simulink model "Clase26112020"  (R2020b)
settings: Solver=VariableStepAuto  StartTime=0.0  StopTime=2  RelTol=1e-3
libraries: dspvision x2, commanapbnd3 x1
settings Model: Creator=fernando  LastModifiedBy=fernando

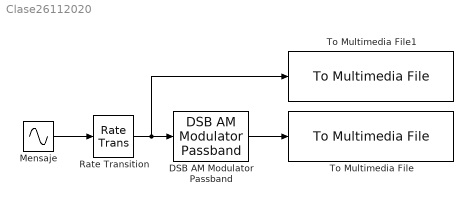
== system Clase26112020 ==
  DSB AM Modulator Passband : commanapbnd3/DSB AM Modulator Passband  Fc=10E3  Ph=0  Offset=1
      settings: SourceProductBaseCode=CM
  Mensaje : Sin  Frequency=2*pi*440  SampleTime=0
  Rate Transition : RateTransition  OutPortSampleTime=1/44100
  To Multimedia File : dspvision/To Multimedia File  outputFilename=SalidaModulada.wav  streamSelection=Audio only  videoCompressor=None (uncompressed)  audioCompressor=None (uncompressed)  imagePorts=Separate color signals  fileType=WAV  audioDatatype=16-bit integer  fourcc=RGB  videoQuality=75  mj2000CompFactor=10
  To Multimedia File1 : dspvision/To Multimedia File  outputFilename=SalidaNoModulada.wav  streamSelection=Audio only  videoCompressor=None (uncompressed)  audioCompressor=None (uncompressed)  imagePorts=Separate color signals  fileType=WAV  audioDatatype=16-bit integer  fourcc=RGB  videoQuality=75  mj2000CompFactor=10
  wires:
  Mensaje/1 -> Rate Transition/1
  Rate Transition/1 -> To Multimedia File1/1, DSB AM Modulator Passband/1
  DSB AM Modulator Passband/1 -> To Multimedia File/1
